simulink model "minimal_smib_discrete"  (R2025b)
settings: Solver=FixedStepAuto  StartTime=0.0  StopTime=5  FixedStep=50e-6  RelTol=1e-3
undefined symbols (not defined in the file or in its folder): D_vsg, LoadStep_t_s, M_vsg, Pm_pu_vsg
libraries: spsControlledVoltageSourceLib x3, spsSeriesRLCBranchLib x3, spsThreePhaseSeriesRLCLoadLib x2, spsThreePhaseBreakerLib x1, spsGroundLib x1, spsThreePhaseVIMeasurementLib x1, spspowerguiLib x1
settings Model: Creator=27443  LastModifiedBy=27443

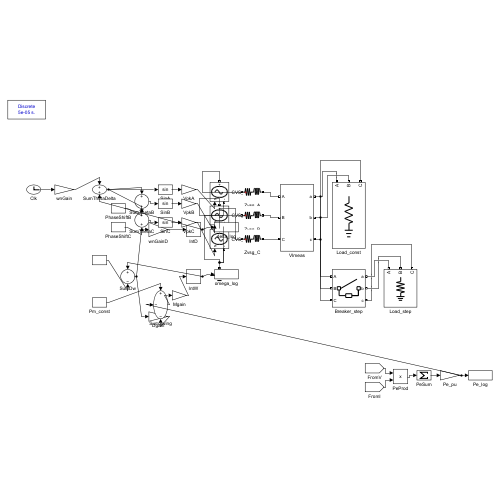
[thumbnail: Simulink's stored preview of the top-level diagram]
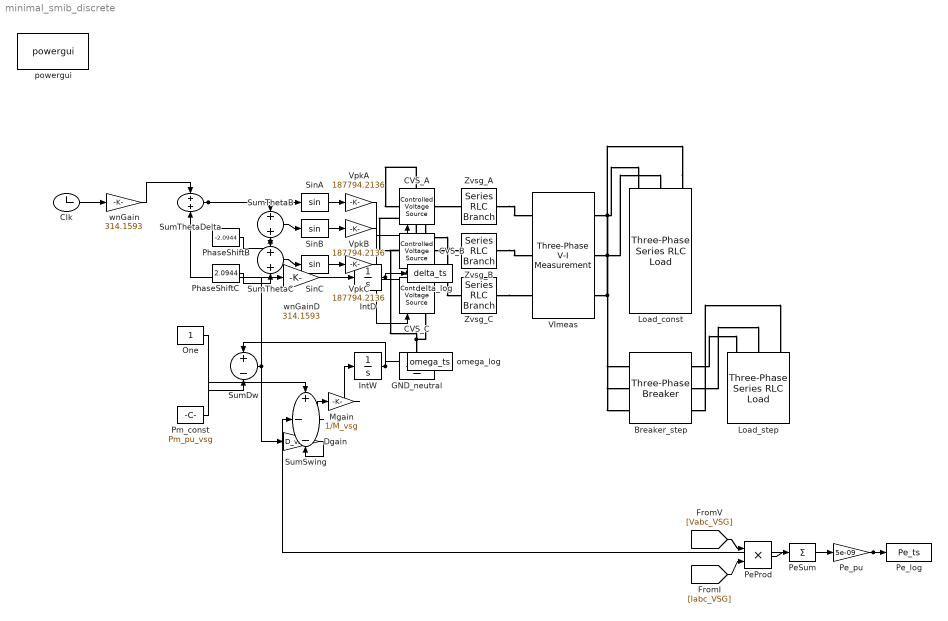
== system minimal_smib_discrete ==
  Breaker_step : spsThreePhaseBreakerLib/Three-Phase Breaker  InitialState=open  SwitchA=on  SwitchB=on  SwitchC=on  SwitchTimes=[LoadStep_t_s]  External=off  BreakerResistance=0.01  SnubberResistance=1e6  SnubberCapacitance=inf  Measurements=None
  CVS_A : spsControlledVoltageSourceLib/Controlled Voltage Source  Initialize=on  Source_Type=AC  Amplitude=0  Phase=0  Frequency=0  Measurements=None
  CVS_B : spsControlledVoltageSourceLib/Controlled Voltage Source  Initialize=on  Source_Type=AC  Amplitude=0  Phase=0  Frequency=0  Measurements=None
  CVS_C : spsControlledVoltageSourceLib/Controlled Voltage Source  Initialize=on  Source_Type=AC  Amplitude=0  Phase=0  Frequency=0  Measurements=None
  Clk : Clock
  Dgain : Gain  Gain=D_vsg
  GND_neutral : spsGroundLib/Ground  LConnTagsString=a
  IntD : Integrator
  IntW : Integrator  InitialCondition=1
  Load_const : spsThreePhaseSeriesRLCLoadLib/Three-Phase Series RLC Load  LConnTagsString=A|B|C  Configuration=Y (grounded)  NominalVoltage=230000  Vabc=[1e3 1e3 1e3]  Vabcp=[1e3 1e3 1e3]  NominalFrequency=50  UnbalancedPower=off  ActivePower=40000000  InductivePower=0  CapacitivePower=0  Pabc=[10e3 9e3 11e3]  QLabc=[100 90 110]  QCabc=[100 90 110]  Pabcp=[10e3 9e3 11e3]  QLabcp=[100 90 110]  QCabcp=[100 90 110]  Measurements=None  LoadType=constant Z
  Load_step : spsThreePhaseSeriesRLCLoadLib/Three-Phase Series RLC Load  LConnTagsString=A|B|C  Configuration=Y (grounded)  NominalVoltage=230000  Vabc=[1e3 1e3 1e3]  Vabcp=[1e3 1e3 1e3]  NominalFrequency=50  UnbalancedPower=off  ActivePower=LoadStep_amp_W  InductivePower=0  CapacitivePower=0  Pabc=[10e3 9e3 11e3]  QLabc=[100 90 110]  QCabc=[100 90 110]  Pabcp=[10e3 9e3 11e3]  QLabcp=[100 90 110]  QCabcp=[100 90 110]  Measurements=None  LoadType=constant Z
  Mgain : Gain  Gain=1/M_vsg
  One : Constant
  PeProd : Product
  PeSum : Sum  Inputs=+
  Pe_log : ToWorkspace  VariableName=Pe_ts  SaveFormat=Timeseries  SampleTime=-1
  Pe_pu : Gain  Gain=5e-09
  PhaseShiftB : Constant  Value=-2.0944
  PhaseShiftC : Constant  Value=2.0944
  Pm_const : Constant  Value=Pm_pu_vsg
  SinA : Trigonometry
  SinB : Trigonometry
  SinC : Trigonometry
  SumDw : Sum  Inputs=+-
  SumSwing : Sum  Inputs=+--
  SumThetaB : Sum
  SumThetaC : Sum
  SumThetaDelta : Sum
  VImeas : spsThreePhaseVIMeasurementLib/Three-Phase V-I Measurement  VoltageMeasurement=phase-to-ground  SetLabelV=on  LabelV=Vabc_VSG  Vpu=off  VpuLL=off  CurrentMeasurement=yes  SetLabelI=on  LabelI=Iabc_VSG  Ipu=off  Pbase=100e6  Vbase=500e3  OutputType=Complex  PhasorSimulation=off  PSBequivalent=0
  VpkA : Gain  Gain=187794.2136
  VpkB : Gain  Gain=187794.2136
  VpkC : Gain  Gain=187794.2136
  Zvsg_A : spsSeriesRLCBranchLib/Series RLC Branch  LConnTagsString=__new0  RConnTagsString=__new0  BranchType=RL  Resistance=0.7935  Inductance=0.25258  SetiL0=off  InitialCurrent=0  Capacitance=1e-6  Setx0=off  InitialVoltage=0  Measurements=None
  Zvsg_B : spsSeriesRLCBranchLib/Series RLC Branch  LConnTagsString=__new0  RConnTagsString=__new0  BranchType=RL  Resistance=0.7935  Inductance=0.25258  SetiL0=off  InitialCurrent=0  Capacitance=1e-6  Setx0=off  InitialVoltage=0  Measurements=None
  Zvsg_C : spsSeriesRLCBranchLib/Series RLC Branch  LConnTagsString=__new0  RConnTagsString=__new0  BranchType=RL  Resistance=0.7935  Inductance=0.25258  SetiL0=off  InitialCurrent=0  Capacitance=1e-6  Setx0=off  InitialVoltage=0  Measurements=None
  delta_log : ToWorkspace  VariableName=delta_ts  SaveFormat=Timeseries  SampleTime=-1
  omega_log : ToWorkspace  VariableName=omega_ts  SaveFormat=Timeseries  SampleTime=-1
  powergui : spspowerguiLib/powergui  Priority=1  SimulationMode=Discrete  SampleTime=50e-6  frequency=60  Iterations=50  frequencyindice=60  Pbase=100e6  ErrMax=1e-4  UnitsV=kV  UnitsW=MW  buscounter=0  FunctionMessages=off  echomessages=off  EnableUseOfTLC=off  CurrentSourceSwitches=off  DisableSnubberDevices=off  DisableRonSwitches=off  DisableVfSwitches=off  DisplayEquations=off  AutomaticDiscreteSolvers=off  SolverType=Tustin/Backward Euler (TBE)  Interpol=off  ExternalGateDelay=off  methode=off  Ts=100  x0status=blocks  SPID=on  SwTol=0  HookPort=off  NonlinearTolerance=1e-4  nMaxIteration=100  ContinueOnMaxIteration=off  RestoreLinks=warning  ResistiveCurrentMeasurement=off  Frange=[0:2:500]  Ylog=off  Xlog=on  ShowGrid=off  save=off  variable=ZData  structure=0  ZoomFFT=off  StartTime=0.0  cycles=1  DisplayStyle=1  fundamental=60  FreqAxis=off  MaxFrequency=1000  frequencyindicesteady=1  RmsSteady=1  display=off
  wnGain : Gain  Gain=314.1593
  wnGainD : Gain  Gain=314.1593
  wires:
  Clk/1 -> wnGain/1
  wnGain/1 -> SumThetaDelta/1
  IntW/1 -> SumDw/1, omega_log/1
  One/1 -> SumDw/2
  SumDw/1 -> wnGainD/1, Dgain/1
  wnGainD/1 -> IntD/1
  IntD/1 -> SumThetaDelta/2, delta_log/1
  SumThetaDelta/1 -> SumThetaB/1, SumThetaC/1, SinA/1
  PhaseShiftB/1 -> SumThetaB/2
  PhaseShiftC/1 -> SumThetaC/2
  SumThetaB/1 -> SinB/1
  SumThetaC/1 -> SinC/1
  SinA/1 -> VpkA/1
  SinB/1 -> VpkB/1
  SinC/1 -> VpkC/1
  VpkA/1 -> CVS_A/1
  VpkB/1 -> CVS_B/1
  VpkC/1 -> CVS_C/1
  [Vabc_VSG] -> PeProd/1
  [Iabc_VSG] -> PeProd/2
  PeProd/1 -> PeSum/1
  PeSum/1 -> Pe_pu/1
  Pe_pu/1 -> Pe_log/1, SumSwing/2
  Pm_const/1 -> SumSwing/1
  Dgain/1 -> SumSwing/3
  SumSwing/1 -> Mgain/1
  Mgain/1 -> IntW/1
  connections:
  CVS_A/LConn1 -- CVS_B/LConn1 -- GND_neutral/LConn1 -- CVS_C/LConn1
  CVS_A/RConn1 -- Zvsg_A/LConn1
  CVS_B/RConn1 -- Zvsg_B/LConn1
  CVS_C/RConn1 -- Zvsg_C/LConn1
  Zvsg_A/RConn1 -- VImeas/LConn1
  Zvsg_B/RConn1 -- VImeas/LConn2
  Zvsg_C/RConn1 -- VImeas/LConn3
  Load_const/LConn1 -- VImeas/RConn1 -- Breaker_step/LConn1
  Load_const/LConn2 -- VImeas/RConn2 -- Breaker_step/LConn2
  Load_const/LConn3 -- VImeas/RConn3 -- Breaker_step/LConn3
  Breaker_step/RConn1 -- Load_step/LConn1
  Breaker_step/RConn2 -- Load_step/LConn2
  Breaker_step/RConn3 -- Load_step/LConn3
